simulink model "u2dd_ml"  (R2023a)
settings: Solver=VariableStepAuto  StartTime=0.0  StopTime=10.0  RelTol=1e-3
settings Model: Creator=Boss  LastModifiedBy=Boss

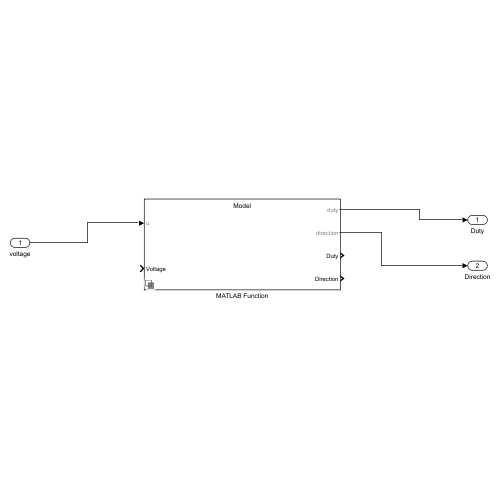
[thumbnail: Simulink's stored preview of the top-level diagram]
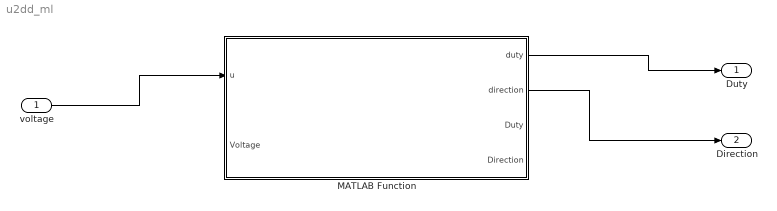
== system u2dd_ml ==
  voltage : Inport
  MATLAB Function : Subsystem  Variant=on  VariantControlMode=label  VariantControl=Choice  LabelModeActiveChoice=Choice_1
  Duty : Outport
  Direction : Outport  Port=2
  wires:
  voltage/1 -> MATLAB Function/1(u)
  MATLAB Function/1(duty) -> Duty/1
  MATLAB Function/2(direction) -> Direction/1

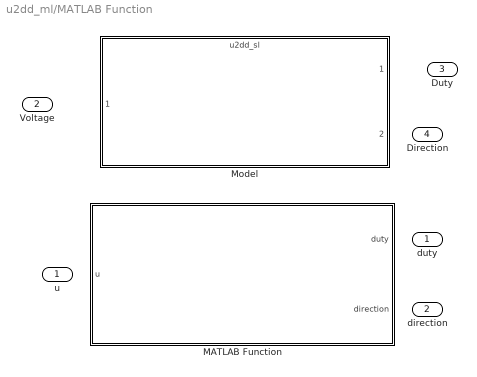
== system u2dd_ml/MATLAB Function ==
  u : Inport
  Voltage : Inport  Port=2
  MATLAB Function : MATLAB Function  TreatAsAtomicUnit=on  VariantControl=Choice
  Model : ModelReference  ModelNameDialog=u2dd_sl.slx  SimulationMode=Normal  VariantControl=Choice_1  ModelReferenceVersion=1.1
  duty : Outport
  direction : Outport  Port=2
  Duty : Outport  Port=3
  Direction : Outport  Port=4

== matlab function u2dd_ml/MATLAB Function/MATLAB Function ==
  data: u input; duty output; direction output
function [duty, direction] = u2dd(u)

% direção do bit e conifguração do duty = abs(u)
if u >= 0
    duty = u;
    direction = 1;
else
    duty = -u;
    direction = -1;
end

% Saturação do duty cycle a 1
if duty > 1
    duty = 1;
end
